simulink model "timetriggered"  (Simulink 4.00)
settings: Solver=ode45  StartTime=0.0  StopTime=10  RelTol=1e-3
InitFcn:
  | clear functions
libraries: truetime x5, simulink3 x1
settings Model: Creator=anton  LastModifiedBy=anton  OutputTimes=[0.00199]  SaveTime=off  SaveOutput=off  LimitDataPoints=off  RTWOptions="-aEnforceIntegerDowncast=1 -aExtMode=0 -aFoldNonRolledExpr=1 -aForceParamTrailComments=0 -aGenerateComments=1 -aIgnoreCustomStorageClasses=0 -aIncHierarchyInIds=0 -aInlineInvariantSignals=0 -aLocalBlockOutputs=1 -aLogVarNameModifier=\"rt_\" -aRTWVerbose=1 -aRollThreshold=5 -aShowEliminatedStatements=1"  ExtModeTrigMode=oneshot  ExtModeArmWhenConnect=off  ExtModeAutoUpdateStatusClock=off  BlockReductionOpt=off

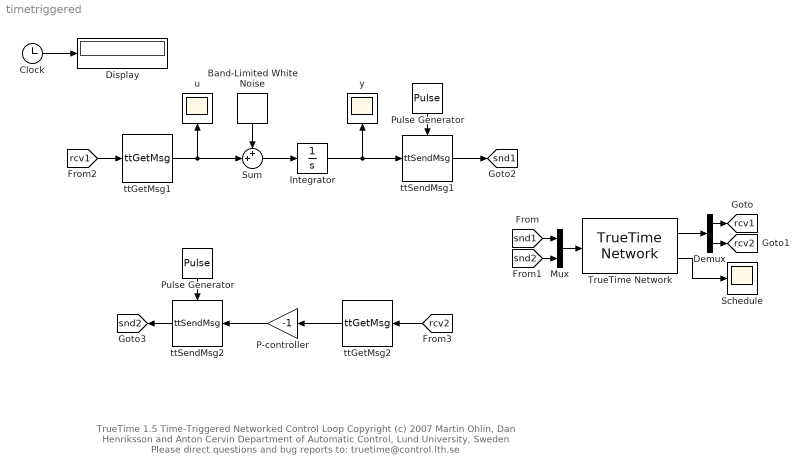
== system timetriggered ==
  note: TrueTime 1.5  Time-Triggered Networked Control Loop
      | Copyright (c) 2007
      | Martin Ohlin, Dan Henriksson and Anton Cervin
      | Department of Automatic Control, Lund University, Sweden
      | Please direct questions and bug reports to:  truetime@control.lth.se
  Band-Limited White Noise : simulink3/Sources/Band-Limited White Noise  Orientation=down  Cov=[0.1]  Ts=0.1  seed=[23341]
  Clock : Clock
      settings: DisplayTime=off  Decimation=10
  Demux : Demux  Outputs=2  BusSelectionMode=off
  Display : Display
      settings: Format=short
  Integrator : Integrator  ExternalReset=none  InitialConditionSource=internal  InitialCondition=0  LimitOutput=off  UpperSaturationLimit=inf  LowerSaturationLimit=-inf  ShowSaturationPort=off  ShowStatePort=off  AbsoluteTolerance=auto
  Mux : Mux  Inputs=2
  P-controller : Gain  Orientation=left  Gain=-1  Multiplication=Element-wise(K.*u)  SaturateOnIntegerOverflow=on
  Pulse Generator : DiscretePulseGenerator  Orientation=down  PulseType=Time-based  Amplitude=1  Period=0.1  PulseWidth=50  PhaseDelay=0  SampleTime=1
  "Pulse Generator " : DiscretePulseGenerator  Orientation=down  PulseType=Time-based  Amplitude=1  Period=0.1  PulseWidth=50  PhaseDelay=0.05  SampleTime=1
  Schedule : Scope
      settings: TimeRange=10  YMin=1  YMax=2.5  SaveToWorkspace=off  SaveName=ScopeData  MaxDataPoints=5000
  Sum : Sum  Inputs=++|  SaturateOnIntegerOverflow=on
  TrueTime Network : truetime/TrueTime Network  nwtype=CSMA/CD (Ethernet)  nwnbr=1  nnodes=2  rate=10000000  minsize=512  lossprob=0  bandwidths=[0.5 0.5]  slotsize=512  schedule=[1 1 2]  memsize=80000  buftype=Common buffer  overflow=Retransmit
  ttGetMsg1 : truetime/ttGetMsg  network=1  receiver=1  trigger=off
  ttGetMsg2 : truetime/ttGetMsg  Orientation=left  network=1  receiver=2  trigger=off
  ttSendMsg1 : truetime/ttSendMsg  Priority=1  network=1  network_input=off  sender=1  sender_input=off  receiver=2  receiver_input=off  data=0  data_input=on  length=1000  length_input=off  priority=1  priority_input=off  TriggerType=rising
  ttSendMsg2 : truetime/ttSendMsg  Orientation=left  Priority=1  network=1  network_input=off  sender=2  sender_input=off  receiver=1  receiver_input=off  data=0  data_input=on  length=1000  length_input=off  priority=1  priority_input=off  TriggerType=rising
  u : Scope
      settings: Orientation=up  TimeRange=10  YMin=-1  YMax=1  SaveToWorkspace=off  SaveName=ScopeData2  LimitDataPoints=on  MaxDataPoints=5000
  y : Scope
      settings: Orientation=up  TimeRange=10  YMin=-1  YMax=1  SaveToWorkspace=off  MaxDataPoints=5000
  tag scope: rcv1=global, rcv2=global, snd1=global, snd2=global
  wires:
  Clock/1 -> Display/1
  Integrator/1 -> ttSendMsg1/1, y/1
  Pulse Generator/1 -> ttSendMsg1/Trigger
  ttSendMsg1/1 -> [snd1]
  TrueTime Network/1 -> Demux/1
  [snd2] -> Mux/2
  [snd1] -> Mux/1
  Demux/1 -> [rcv1]
  Demux/2 -> [rcv2]
  TrueTime Network/2 -> Schedule/1
  ttGetMsg2/1 -> P-controller/1
  P-controller/1 -> ttSendMsg2/1
  ttSendMsg2/1 -> [snd2]
  [rcv1] -> ttGetMsg1/1
  [rcv2] -> ttGetMsg2/1
  "Pulse Generator "/1 -> ttSendMsg2/Trigger
  Mux/1 -> TrueTime Network/1
  Sum/1 -> Integrator/1
  Band-Limited White Noise/1 -> Sum/1
  ttGetMsg1/1 -> Sum/2, u/1
